simulink model "switch_case"  (R2021a)
settings: Solver=VariableStepAuto  StartTime=0.0  StopTime=10.0  RelTol=1e-3
settings Model: Creator=reemb  LastModifiedBy=reemb

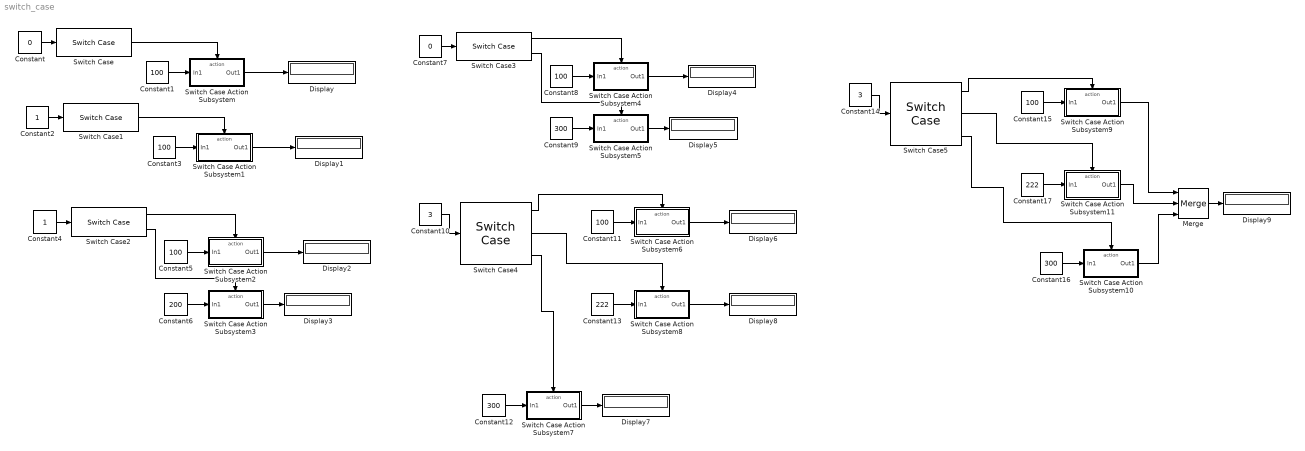
== system switch_case ==
  Constant : Constant  Value=0
  Constant{1,3,5,8,11,15} (6 alike) : Constant  Value=100
  Constant10 : Constant  Value=3
  Constant12 : Constant  Value=300
  Constant13 : Constant  Value=222
  Constant14 : Constant  Value=3
  Constant16 : Constant  Value=300
  Constant17 : Constant  Value=222
  Constant2 : Constant
  Constant4 : Constant
  Constant6 : Constant  Value=200
  Constant7 : Constant  Value=0
  Constant9 : Constant  Value=300
  Display{,1..9} (10 alike) : Display
  Merge : Merge  Inputs=3
  Switch Case : SwitchCase  ShowDefaultCase=off
  Switch Case Action Subsystem : Subsystem  TreatAsAtomicUnit=on
  Switch Case Action Subsystem1 : Subsystem  TreatAsAtomicUnit=on
  Switch Case Action Subsystem10 : Subsystem  TreatAsAtomicUnit=on
  Switch Case Action Subsystem11 : Subsystem  TreatAsAtomicUnit=on
  Switch Case Action Subsystem2 : Subsystem  TreatAsAtomicUnit=on
  Switch Case Action Subsystem3 : Subsystem  TreatAsAtomicUnit=on
  Switch Case Action Subsystem4 : Subsystem  TreatAsAtomicUnit=on
  Switch Case Action Subsystem5 : Subsystem  TreatAsAtomicUnit=on
  Switch Case Action Subsystem6 : Subsystem  TreatAsAtomicUnit=on
  Switch Case Action Subsystem7 : Subsystem  TreatAsAtomicUnit=on
  Switch Case Action Subsystem8 : Subsystem  TreatAsAtomicUnit=on
  Switch Case Action Subsystem9 : Subsystem  TreatAsAtomicUnit=on
  Switch Case1 : SwitchCase  ShowDefaultCase=off
  Switch Case2 : SwitchCase  CaseConditions={1,2}  ShowDefaultCase=off
  Switch Case3 : SwitchCase
  Switch Case4 : SwitchCase  CaseConditions={1,[2 3]}
  Switch Case5 : SwitchCase  CaseConditions={1,[2 3]}
  wires:
  Switch Case Action Subsystem/1(Out1) -> Display/1
  Switch Case/1 -> Switch Case Action Subsystem/Action
  Constant/1 -> Switch Case/1
  Constant1/1 -> Switch Case Action Subsystem/1(In1)
  Constant3/1 -> Switch Case Action Subsystem1/1(In1)
  Constant2/1 -> Switch Case1/1
  Switch Case1/1 -> Switch Case Action Subsystem1/Action
  Switch Case Action Subsystem1/1(Out1) -> Display1/1
  Switch Case Action Subsystem2/1(Out1) -> Display2/1
  Switch Case2/1 -> Switch Case Action Subsystem2/Action
  Constant4/1 -> Switch Case2/1
  Constant5/1 -> Switch Case Action Subsystem2/1(In1)
  Constant6/1 -> Switch Case Action Subsystem3/1(In1)
  Switch Case2/2 -> Switch Case Action Subsystem3/Action
  Switch Case Action Subsystem3/1(Out1) -> Display3/1
  Switch Case Action Subsystem5/1(Out1) -> Display5/1
  Switch Case3/2 -> Switch Case Action Subsystem5/Action
  Constant9/1 -> Switch Case Action Subsystem5/1(In1)
  Constant8/1 -> Switch Case Action Subsystem4/1(In1)
  Constant7/1 -> Switch Case3/1
  Switch Case3/1 -> Switch Case Action Subsystem4/Action
  Switch Case Action Subsystem4/1(Out1) -> Display4/1
  Switch Case Action Subsystem6/1(Out1) -> Display6/1
  Switch Case4/1 -> Switch Case Action Subsystem6/Action
  Constant10/1 -> Switch Case4/1
  Constant11/1 -> Switch Case Action Subsystem6/1(In1)
  Constant12/1 -> Switch Case Action Subsystem7/1(In1)
  Switch Case4/3 -> Switch Case Action Subsystem7/Action
  Switch Case Action Subsystem7/1(Out1) -> Display7/1
  Constant13/1 -> Switch Case Action Subsystem8/1(In1)
  Switch Case Action Subsystem8/1(Out1) -> Display8/1
  Switch Case4/2 -> Switch Case Action Subsystem8/Action
  Switch Case5/2 -> Switch Case Action Subsystem11/Action
  Switch Case Action Subsystem11/1(Out1) -> Merge/2
  Constant17/1 -> Switch Case Action Subsystem11/1(In1)
  Switch Case Action Subsystem10/1(Out1) -> Merge/3
  Switch Case5/3 -> Switch Case Action Subsystem10/Action
  Constant16/1 -> Switch Case Action Subsystem10/1(In1)
  Constant15/1 -> Switch Case Action Subsystem9/1(In1)
  Constant14/1 -> Switch Case5/1
  Switch Case5/1 -> Switch Case Action Subsystem9/Action
  Merge/1 -> Display9/1
  Switch Case Action Subsystem9/1(Out1) -> Merge/1

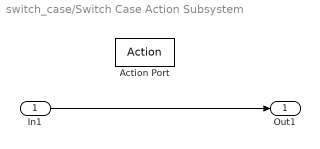
== system switch_case/Switch Case Action Subsystem ==
  In1 : Inport
  Action Port : ActionPort  ActionPortLabel=case [ 1 ]:
  Out1 : Outport
  wires:
  In1/1 -> Out1/1

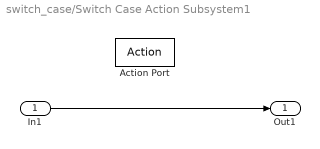
== system switch_case/Switch Case Action Subsystem1 ==
  In1 : Inport
  Action Port : ActionPort  ActionPortLabel=case [ 1 ]:
  Out1 : Outport
  wires:
  In1/1 -> Out1/1

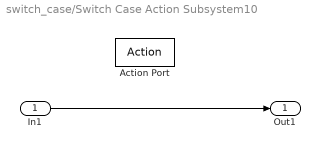
== system switch_case/Switch Case Action Subsystem10 ==
  In1 : Inport
  Action Port : ActionPort  ActionPortLabel=default:
  Out1 : Outport
  wires:
  In1/1 -> Out1/1

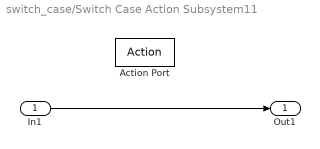
== system switch_case/Switch Case Action Subsystem11 ==
  In1 : Inport
  Action Port : ActionPort  ActionPortLabel=case [ 2 3 ]:
  Out1 : Outport
  wires:
  In1/1 -> Out1/1

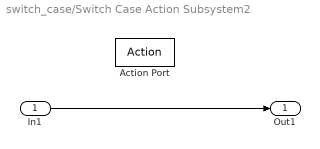
== system switch_case/Switch Case Action Subsystem2 ==
  In1 : Inport
  Action Port : ActionPort  ActionPortLabel=case [ 1 ]:
  Out1 : Outport
  wires:
  In1/1 -> Out1/1

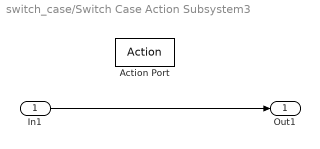
== system switch_case/Switch Case Action Subsystem3 ==
  In1 : Inport
  Action Port : ActionPort  ActionPortLabel=case [ 2 ]:
  Out1 : Outport
  wires:
  In1/1 -> Out1/1

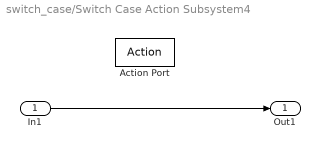
== system switch_case/Switch Case Action Subsystem4 ==
  In1 : Inport
  Action Port : ActionPort  ActionPortLabel=case [ 1 ]:
  Out1 : Outport
  wires:
  In1/1 -> Out1/1

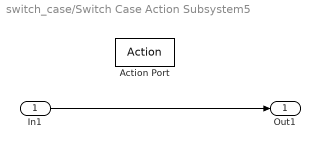
== system switch_case/Switch Case Action Subsystem5 ==
  In1 : Inport
  Action Port : ActionPort  ActionPortLabel=default:
  Out1 : Outport
  wires:
  In1/1 -> Out1/1

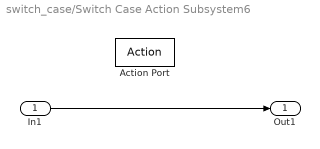
== system switch_case/Switch Case Action Subsystem6 ==
  In1 : Inport
  Action Port : ActionPort  ActionPortLabel=case [ 1 ]:
  Out1 : Outport
  wires:
  In1/1 -> Out1/1

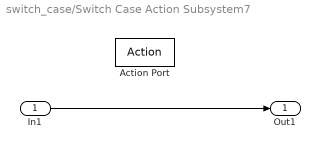
== system switch_case/Switch Case Action Subsystem7 ==
  In1 : Inport
  Action Port : ActionPort  ActionPortLabel=default:
  Out1 : Outport
  wires:
  In1/1 -> Out1/1

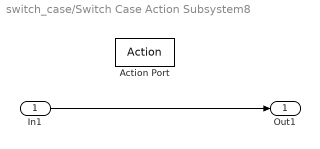
== system switch_case/Switch Case Action Subsystem8 ==
  In1 : Inport
  Action Port : ActionPort  ActionPortLabel=case [ 2 3 ]:
  Out1 : Outport
  wires:
  In1/1 -> Out1/1

== system switch_case/Switch Case Action Subsystem9 ==
  In1 : Inport
  Action Port : ActionPort  ActionPortLabel=case [ 1 ]:
  Out1 : Outport
  wires:
  In1/1 -> Out1/1
